simulink model "Motor_dq_2016a"  (R2016a)
settings: Solver=VariableStepAuto  SolverMode=SingleTasking  StartTime=0.0  StopTime=10  MaxStep=1e-4  RelTol=1e-4
values from neighbouring files (symbols this model uses):
  J = 0.01    [run.m]
  LM = 1.0122e-3    (= 0.0010122)    [run.m]    (also in run_to_complete.m)
  LMatrix = [LS 0 LM 0; 0 LS 0 LM; LM 0 LR 0; 0 LM 0 LR]    [run.m]    (also in run_to_complete.m)
  pp = 2    [run.m]    (also in run_to_complete.m)
  RLInv = RMatrix/(LMatrix)    [run.m]    (also in run_to_complete.m)
settings Model: Creator=João Fernandes  LastModifiedBy=João Fernandes
settings DebuggingCC: SFUnexpectedBacktrackingDiag=error  SFNoUnconditionalDefaultTransitionDiag=error
settings GRTTargetCC: TargetLangStandard=C99 (ISO)  GeneratePreprocessorConditionals=Use local settings
settings ConfigComp: CovMetricSettings=dwe  CovHtmlReporting=off  CovSaveCumulativeToWorkspaceVar=off  CovSaveSingleToWorkspaceVar=off  CovExternalEMLEnable=on

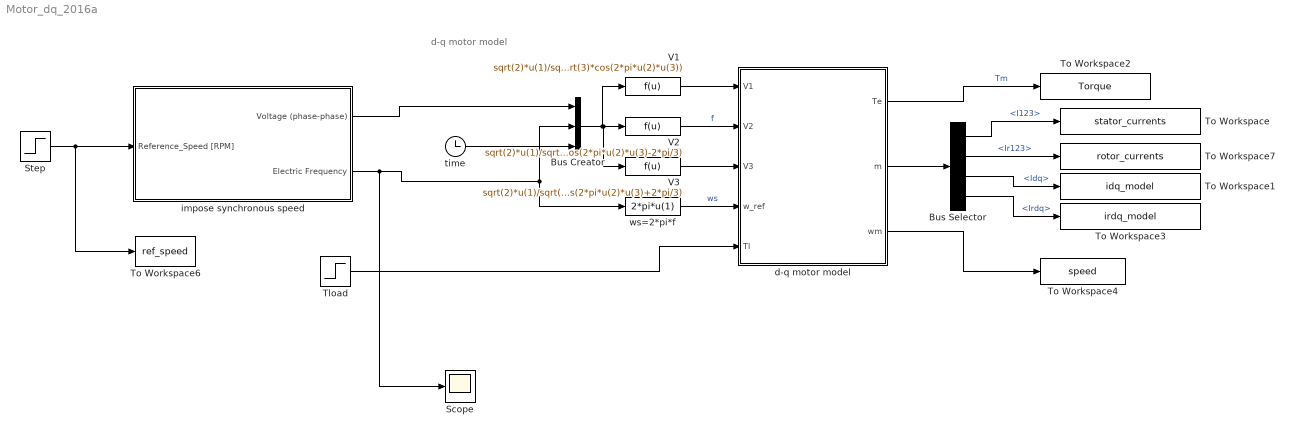
== system Motor_dq_2016a ==
  note: d-q motor model
  Bus Creator : BusCreator  Inputs=3
  Bus Selector : BusSelector  OutputSignals=I123,Ir123,Idq,Irdq
  Scope : Scope
  Step : Step  After=3750  SampleTime=0
  "Tload " : Step  Time=5  After=40  SampleTime=0
  To Workspace : ToWorkspace  VariableName=stator_currents  SaveFormat=Timeseries  SampleTime=-1
  To Workspace1 : ToWorkspace  VariableName=idq_model  SaveFormat=Timeseries  SampleTime=-1
  To Workspace2 : ToWorkspace  VariableName=Torque  SaveFormat=Timeseries  SampleTime=-1
  To Workspace3 : ToWorkspace  VariableName=irdq_model  SaveFormat=Timeseries  SampleTime=-1
  To Workspace4 : ToWorkspace  VariableName=speed  SaveFormat=Timeseries  SampleTime=-1
  To Workspace6 : ToWorkspace  VariableName=ref_speed  SaveFormat=Timeseries  SampleTime=-1
  To Workspace7 : ToWorkspace  VariableName=rotor_currents  SaveFormat=Timeseries  SampleTime=-1
  V1 : Fcn  Expr=sqrt(2)*u(1)/sqrt(3)*cos(2*pi*u(2)*u(3))
  V2 : Fcn  Expr=sqrt(2)*u(1)/sqrt(3)*cos(2*pi*u(2)*u(3)-2*pi/3)
  V3 : Fcn  Expr=sqrt(2)*u(1)/sqrt(3)*cos(2*pi*u(2)*u(3)+2*pi/3)
  d-q motor model : Subsystem
  impose synchronous speed : Subsystem
  time : Clock
  ws=2*pi*f : Fcn  Expr=2*pi*u(1)
  wires:
  V1/1 -> d-q motor model/1(V1)
  ws=2*pi*f/1 -> d-q motor model/4(w_ref)  "ws"
  V2/1 -> d-q motor model/2(V2)  "f"
  d-q motor model/1(Te) -> To Workspace2/1  "Tm"
  Bus Creator/1 -> V1/1, V3/1, V2/1
  time/1 -> Bus Creator/3
  V3/1 -> d-q motor model/3(V3)
  impose synchronous speed/1(Voltage (phase-phase)) -> Bus Creator/1
  impose synchronous speed/2(Electric Frequency) -> Scope/1, Bus Creator/2, ws=2*pi*f/1
  "Tload "/1 -> d-q motor model/5(Tl)
  Step/1 -> To Workspace6/1, impose synchronous speed/1(Reference_Speed [RPM])
  d-q motor model/2(m) -> Bus Selector/1
  Bus Selector/1 -> To Workspace/1  "<I123>"
  Bus Selector/2 -> To Workspace7/1  "<Ir123>"
  d-q motor model/3(wm) -> To Workspace4/1
  Bus Selector/3 -> To Workspace1/1  "<Idq>"
  Bus Selector/4 -> To Workspace3/1  "<Irdq>"

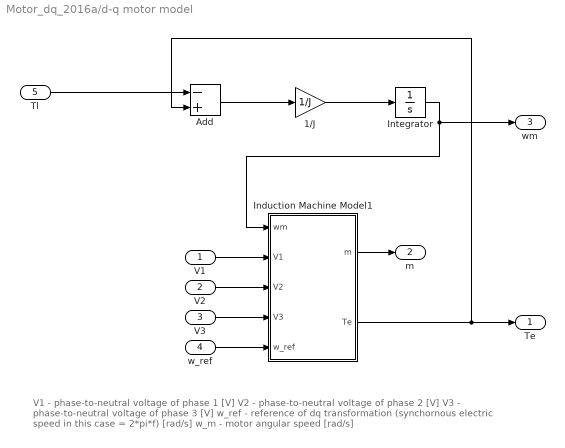
== system Motor_dq_2016a/d-q motor model ==
  note: V1 - phase-to-neutral voltage of phase 1 [V]
      | V2 - phase-to-neutral voltage of phase 2 [V]
      | V3 - phase-to-neutral voltage of phase 3 [V]
      | w_ref - reference of dq transformation (synchornous electric speed in this case = 2*pi*f) [rad/s]
      | w_m - motor angular speed [rad/s]
  V1 : Inport
  V2 : Inport  Port=2
  V3 : Inport  Port=3
  w_ref : Inport  Port=4
  Tl : Inport  Port=5
  1/J : Gain  Gain=1/J
  Add : Sum  Inputs=-+
  Induction Machine Model1 : Subsystem
  Integrator : Integrator
  Te : Outport
  m : Outport  Port=2
  wm : Outport  Port=3
  wires:
  Induction Machine Model1/1(m) -> m/1
  w_ref/1 -> Induction Machine Model1/5(w_ref)
  V1/1 -> Induction Machine Model1/2(V1)
  V2/1 -> Induction Machine Model1/3(V2)
  V3/1 -> Induction Machine Model1/4(V3)
  Integrator/1 -> Induction Machine Model1/1(wm), wm/1
  1/J/1 -> Integrator/1
  Add/1 -> 1/J/1
  Induction Machine Model1/2(Te) -> Add/2, Te/1
  Tl/1 -> Add/1

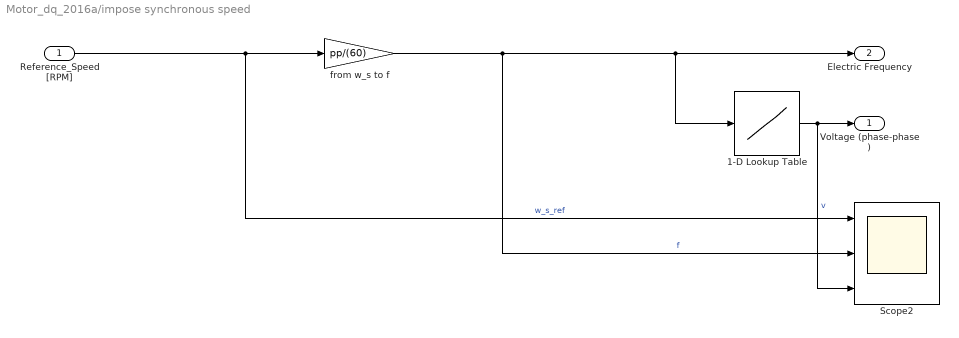
== system Motor_dq_2016a/impose synchronous speed ==
  Reference_Speed [RPM] : Inport
  1-D Lookup Table : Lookup_n-D  NumberOfTableDimensions=1  BreakpointsForDimension1=[0 76 220 305]  Table=[0 76 121 121]  InternalRulePriority=Speed  RndMeth=Simplest  InputSameDT=on
  Scope2 : Scope  NumInputPorts=3
  from w_s to f : Gain  Gain=pp/(60)
  Voltage (phase-phase) : Outport
  Electric Frequency : Outport  Port=2
  wires:
  from w_s to f/1 -> Scope2/2, 1-D Lookup Table/1, Electric Frequency/1  "f"
  1-D Lookup Table/1 -> Scope2/3, Voltage (phase-phase)/1  "v"
  Reference_Speed [RPM]/1 -> Scope2/1, from w_s to f/1  "w_s_ref"

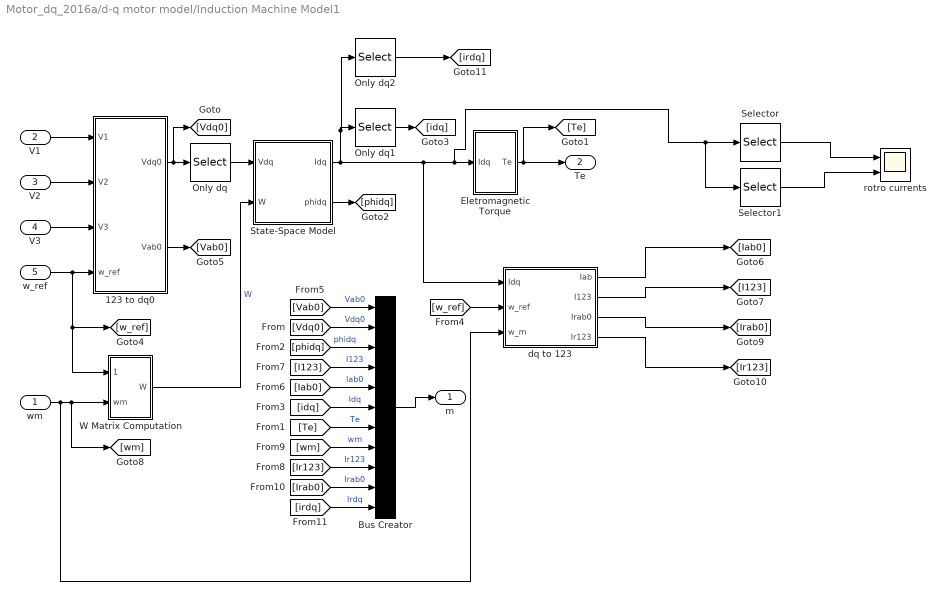
== system Motor_dq_2016a/d-q motor model/Induction Machine Model1 ==
  wm : Inport
  V1 : Inport  Port=2
  V2 : Inport  Port=3
  V3 : Inport  Port=4
  w_ref : Inport  Port=5
  123 to dq0 : Subsystem
  Bus Creator : BusCreator  Inputs=11
  Eletromagnetic Torque : Subsystem
  Only dq : Selector  InputPortWidth=3  IndexOptions=Index vector (dialog)  Indices=[1 2]  OutputSizes=1
  Only dq1 : Selector  InputPortWidth=4  IndexOptions=Index vector (dialog)  Indices=[1 2]  OutputSizes=1
  Only dq2 : Selector  InputPortWidth=4  IndexOptions=Index vector (dialog)  Indices=[3 4]  OutputSizes=1
  Selector : Selector  InputPortWidth=4  IndexOptions=Index vector (dialog)  Indices=[1 2]  OutputSizes=1
  Selector1 : Selector  InputPortWidth=4  IndexOptions=Index vector (dialog)  Indices=[3 4]  OutputSizes=1
  State-Space Model : Subsystem
  W Matrix Computation : Subsystem
  dq to 123 : Subsystem
  rotro currents : Scope  NumInputPorts=2
  m : Outport
  Te : Outport  Port=2
  wires:
  123 to dq0/1(Vdq0) -> Only dq/1, [Vdq0]
  V3/1 -> 123 to dq0/3(V3)
  V2/1 -> 123 to dq0/2(V2)
  wm/1 -> dq to 123/3(w_m), [wm], W Matrix Computation/2(wm)
  123 to dq0/2(Vab0) -> [Vab0]
  W Matrix Computation/1(W) -> State-Space Model/2(W)  "W"
  Only dq/1 -> State-Space Model/1(Vdq)
  Eletromagnetic Torque/1(Te) -> Te/1, [Te]
  V1/1 -> 123 to dq0/1(V1)
  [w_ref] -> dq to 123/2(w_ref)
  State-Space Model/2(phidq) -> [phidq]
  dq to 123/1(Iab) -> [Iab0]
  dq to 123/2(I123) -> [I123]
  [Vab0] -> Bus Creator/1  "Vab0"
  [Vdq0] -> Bus Creator/2  "Vdq0"
  [phidq] -> Bus Creator/3  "phidq"
  [I123] -> Bus Creator/4  "I123"
  [Iab0] -> Bus Creator/5  "Iab0"
  [idq] -> Bus Creator/6  "Idq"
  [Te] -> Bus Creator/7  "Te"
  Bus Creator/1 -> m/1
  Only dq1/1 -> [idq]
  w_ref/1 -> 123 to dq0/4(w_ref), W Matrix Computation/1(w_ref), [w_ref]
  [wm] -> Bus Creator/8  "wm"
  dq to 123/4(Ir123) -> [Ir123]
  dq to 123/3(Irab0) -> [Irab0]
  [Ir123] -> Bus Creator/9  "Ir123"
  [Irab0] -> Bus Creator/10  "Irab0"
  Selector/1 -> rotro currents/1
  Selector1/1 -> rotro currents/2
  State-Space Model/1(Idq) -> dq to 123/1(Idq), Selector1/1, Selector/1, Eletromagnetic Torque/1(Idq), Only dq2/1, Only dq1/1
  Only dq2/1 -> [irdq]
  [irdq] -> Bus Creator/11  "Irdq"

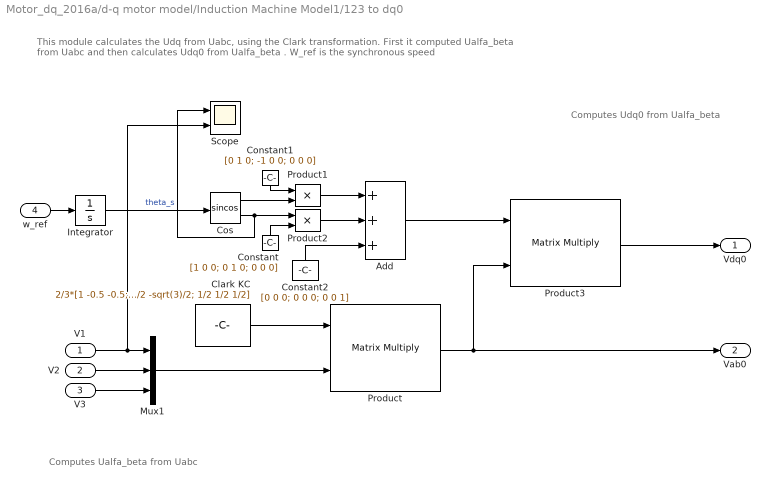
== system Motor_dq_2016a/d-q motor model/Induction Machine Model1/123 to dq0 ==
  note: Computes Ualfa_beta from Uabc
  note: This module calculates the Udq from Uabc, using the Clark transformation.
      | First it computed Ualfa_beta from Uabc and then calculates Udq0 from Ualfa_beta .
      | W_ref is the synchronous speed
  note: Computes Udq0 from Ualfa_beta
  V1 : Inport
  V2 : Inport  Port=2
  V3 : Inport  Port=3
  w_ref : Inport  Port=4
  Add : Sum  Inputs=+++
  Clark KC : Constant  Value=2/3*[1 -0.5 -0.5; 0 sqrt(3)/2 -sqrt(3)/2; 1/2 1/2 1/2]
  Constant : Constant  Value=[1 0 0; 0 1 0; 0 0 0]
  Constant1 : Constant  Value=[0 1 0; -1 0 0; 0 0 0]
  Constant2 : Constant  Value=[0 0 0; 0 0 0; 0 0 1]
  Cos : Trigonometry  Operator=sincos
  Integrator : Integrator
  Mux1 : Mux  Inputs=3
  Product : Product  Multiplication=Matrix(*)
  Product1 : Product
  Product2 : Product
  Product3 : Product  Multiplication=Matrix(*)
  Scope : Scope  NumInputPorts=2
  Vdq0 : Outport
  Vab0 : Outport  Port=2
  wires:
  Clark KC/1 -> Product/1
  Mux1/1 -> Product/2
  Product/1 -> Product3/2, Vab0/1
  Integrator/1 -> Cos/1  "theta_s"
  Cos/1 -> Product1/2
  Constant1/1 -> Product1/1
  Cos/2 -> Scope/1, Product2/1
  Constant/1 -> Product2/2
  Product1/1 -> Add/1
  Product2/1 -> Add/2
  Add/1 -> Product3/1
  Product3/1 -> Vdq0/1
  w_ref/1 -> Integrator/1
  Constant2/1 -> Add/3
  V2/1 -> Mux1/2
  V3/1 -> Mux1/3
  V1/1 -> Mux1/1, Scope/2

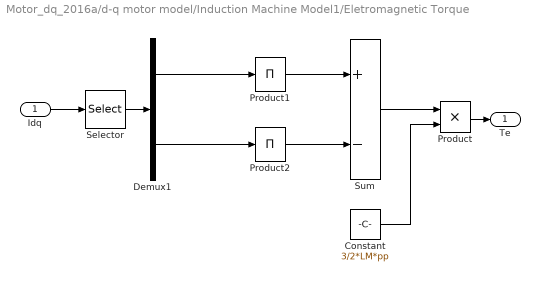
== system Motor_dq_2016a/d-q motor model/Induction Machine Model1/Eletromagnetic Torque ==
  Idq : Inport
  Constant : Constant  Value=3/2*LM*pp
  Demux1 : Demux  Outputs=2
  Product : Product
  Product1 : Product  Inputs=1
  Product2 : Product  Inputs=1
  Selector : Selector  InputPortWidth=4  IndexOptions=Index vector (dialog)  Indices=[2 3 1 4]  OutputSizes=1
  Sum : Sum  Inputs=+-
  Te : Outport
  wires:
  Sum/1 -> Product/1
  Product1/1 -> Sum/1
  Demux1/1 -> Product1/1
  Product2/1 -> Sum/2
  Constant/1 -> Product/2
  Demux1/2 -> Product2/1
  Product/1 -> Te/1
  Idq/1 -> Selector/1
  Selector/1 -> Demux1/1

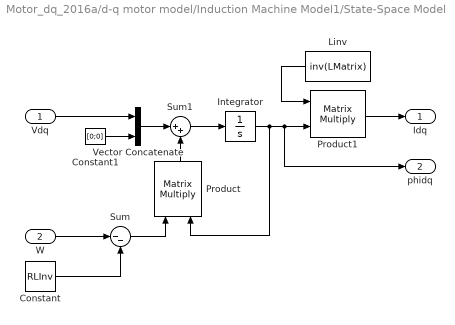
== system Motor_dq_2016a/d-q motor model/Induction Machine Model1/State-Space Model ==
  Vdq : Inport
  W : Inport  Port=2
  Constant : Constant  Value=RLInv  VectorParams1D=off
  Constant1 : Constant  Value=[0;0]
  Integrator : Integrator
  Linv : Constant  Value=inv(LMatrix)  VectorParams1D=off
  Product : Product  Multiplication=Matrix(*)
  Product1 : Product  Multiplication=Matrix(*)
  Sum : Sum  Inputs=|--
  Sum1 : Sum  Inputs=|++
  Vector Concatenate : Concatenate
  Idq : Outport
  phidq : Outport  Port=2
  wires:
  W/1 -> Sum/1
  Product/1 -> Sum1/2
  Constant/1 -> Sum/2
  Integrator/1 -> phidq/1, Product1/2, Product/2
  Product1/1 -> Idq/1
  Sum1/1 -> Integrator/1
  Sum/1 -> Product/1
  Linv/1 -> Product1/1
  Vdq/1 -> Vector Concatenate/1
  Constant1/1 -> Vector Concatenate/2
  Vector Concatenate/1 -> Sum1/1

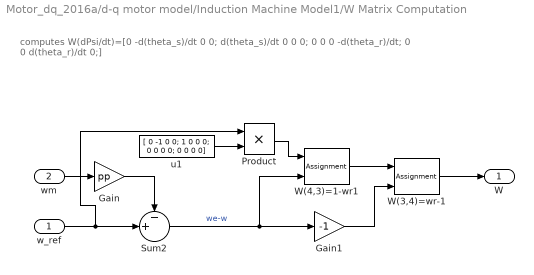
== system Motor_dq_2016a/d-q motor model/Induction Machine Model1/W Matrix Computation ==
  note: computes W(dPsi/dt)=[0                     -d(theta_s)/dt          0                       0;
      |                                     d(theta_s)/dt           0                      0                      0;
      |                                    0                              0                      0             -d(theta_r)/dt;
      |                                    0                              0             d(theta_r)/dt              0;]
  w_ref : Inport
  wm : Inport  Port=2
  Gain : Gain  Gain=pp
  Gain1 : Gain  Gain=-1  SaturateOnIntegerOverflow=on  OutDataTypeStr=Inherit: Same as input  ParamDataTypeStr=Inherit: Same as input
  Product : Product
  Sum2 : Sum  Inputs=-+|  SaturateOnIntegerOverflow=on  InputSameDT=on  OutDataTypeStr=Inherit: Same as first input
  W(3,4)=wr-1 : Assignment  NumberOfDimensions=2  IndexOptions=Index vector (dialog),Index vector (dialog)  Indices=3,4  OutputSizes=1,1
  W(4,3)=1-wr1 : Assignment  NumberOfDimensions=2  IndexOptions=Index vector (dialog),Index vector (dialog)  Indices=4,3  OutputSizes=1,1
  u1 : Constant  Value="[ 0 -1  0  0; 1  0  0  0;  0  0  0  0;  0  0  0  0]"
  W : Outport  InitialOutput=0
  wires:
  Gain1/1 -> W(3,4)=wr-1/2
  W(3,4)=wr-1/1 -> W/1
  Sum2/1 -> W(4,3)=1-wr1/2, Gain1/1  "we-w"
  wm/1 -> Gain/1
  W(4,3)=1-wr1/1 -> W(3,4)=wr-1/1
  Gain/1 -> Sum2/1
  w_ref/1 -> Product/1, Sum2/2
  u1/1 -> Product/2
  Product/1 -> W(4,3)=1-wr1/1

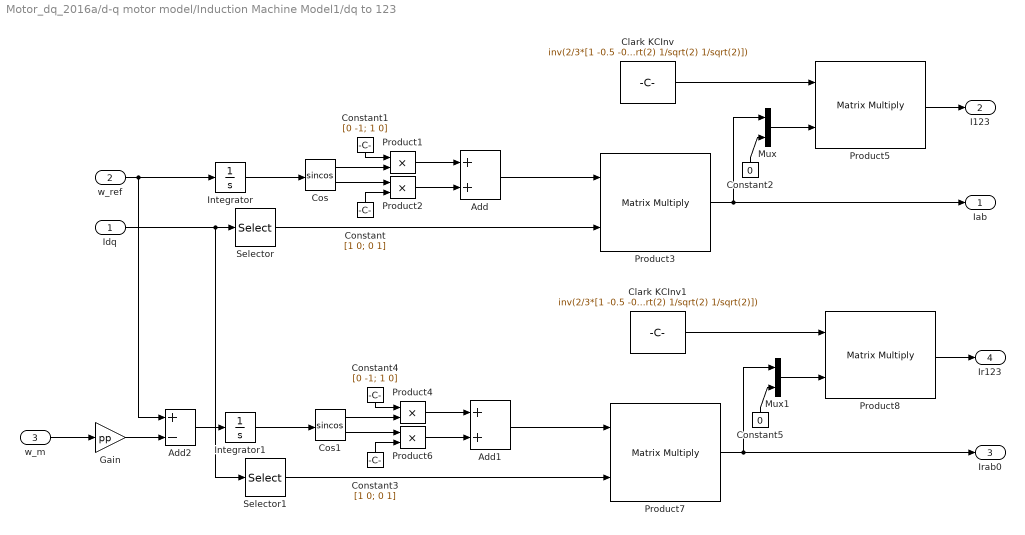
== system Motor_dq_2016a/d-q motor model/Induction Machine Model1/dq to 123 ==
  Idq : Inport
  w_ref : Inport  Port=2
  w_m : Inport  Port=3
  Add : Sum
  Add1 : Sum
  Add2 : Sum  Inputs=+-
  Clark KCInv : Constant  Value=inv(2/3*[1 -0.5 -0.5; 0 sqrt(3)/2 -sqrt(3)/2; 1/sqrt(2) 1/sqrt(2) 1/sqrt(2)])
  Clark KCInv1 : Constant  Value=inv(2/3*[1 -0.5 -0.5; 0 sqrt(3)/2 -sqrt(3)/2; 1/sqrt(2) 1/sqrt(2) 1/sqrt(2)])
  Constant : Constant  Value=[1 0; 0 1]
  Constant1 : Constant  Value=[0 -1; 1 0]
  Constant2 : Constant  Value=0
  Constant3 : Constant  Value=[1 0; 0 1]
  Constant4 : Constant  Value=[0 -1; 1 0]
  Constant5 : Constant  Value=0
  Cos : Trigonometry  Operator=sincos
  Cos1 : Trigonometry  Operator=sincos
  Gain : Gain  Gain=pp
  Integrator : Integrator
  Integrator1 : Integrator
  Mux : Mux  Inputs=2
  Mux1 : Mux  Inputs=2
  Product{1..2,4,6} (4 alike) : Product
  Product{3,5,7..8} (4 alike) : Product  Multiplication=Matrix(*)
  Selector : Selector  InputPortWidth=4  IndexOptions=Index vector (dialog)  Indices=[1 2]  OutputSizes=1
  Selector1 : Selector  InputPortWidth=4  IndexOptions=Index vector (dialog)  Indices=[3 4]  OutputSizes=1
  Iab : Outport
  I123 : Outport  Port=2
  Irab0 : Outport  Port=3
  Ir123 : Outport  Port=4
  wires:
  Cos/1 -> Product1/2
  Constant1/1 -> Product1/1
  Product2/1 -> Add/2
  Cos/2 -> Product2/1
  Product1/1 -> Add/1
  Constant/1 -> Product2/2
  Add/1 -> Product3/1
  Product3/1 -> Mux/1, Iab/1
  Clark KCInv/1 -> Product5/1
  Product5/1 -> I123/1
  Mux/1 -> Product5/2
  Constant2/1 -> Mux/2
  Selector/1 -> Product3/2
  Integrator/1 -> Cos/1
  w_ref/1 -> Integrator/1, Add2/1
  Cos1/1 -> Product4/2
  Selector1/1 -> Product7/2
  Integrator1/1 -> Cos1/1
  Clark KCInv1/1 -> Product8/1
  Constant3/1 -> Product6/2
  Product8/1 -> Ir123/1
  Idq/1 -> Selector1/1, Selector/1
  Cos1/2 -> Product6/1
  Constant4/1 -> Product4/1
  Constant5/1 -> Mux1/2
  Product4/1 -> Add1/1
  Add1/1 -> Product7/1
  Mux1/1 -> Product8/2
  Product6/1 -> Add1/2
  Product7/1 -> Mux1/1, Irab0/1
  w_m/1 -> Gain/1
  Add2/1 -> Integrator1/1
  Gain/1 -> Add2/2
